simulink model "InverseKinematics_DirectionalController2018b"  (R2018b)
settings: Solver=VariableStepAuto  StartTime=0.0  StopTime=inf  RelTol=1e-3
undefined symbols (not defined in the file): f
libraries: instrumentlib x15, dspnetwork x6
(part 1 of 3)
settings Model: Creator=nisit  LastModifiedBy=Jskyl
settings DataIOCC: ReturnWorkspaceOutputs=on

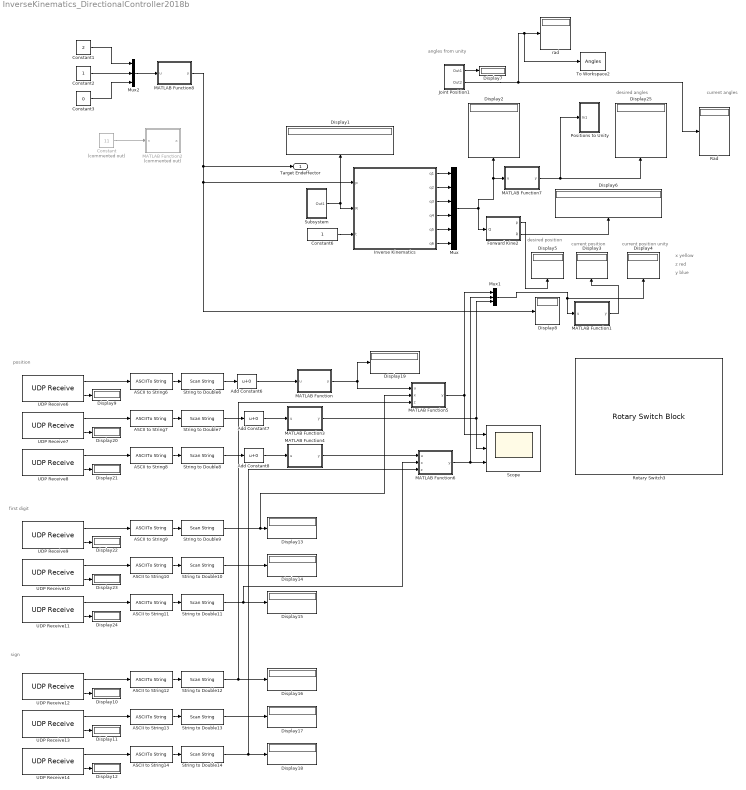
== system InverseKinematics_DirectionalController2018b ==
  note: angles from unity
  note: sign
  note: first digit
  note: position
  note: x yellow
  note: current position unity
  note: current position
  note: desired position
  note: current angles
  note: desired angles
  note: z red
  note: y blue
  ASCII to String{6..14} (9 alike) : ASCIIToString
  Add Constant6 : Bias
  Add Constant7 : Bias
  Add Constant8 : Bias
  Constant : Constant  Commented=on  Value=11
  Constant1 : Constant  Value=2
  Constant2 : Constant
  Constant3 : Constant  Value=0
  Constant6 : Constant
  Display{1..25} (25 alike) : Display
      Display10 settings: Format=bank
      Display11 settings: Format=bank
      Display12 settings: Format=bank
      Display20 settings: Format=bank
      Display21 settings: Format=bank
      Display22 settings: Format=bank
      Display23 settings: Format=bank
      Display24 settings: Format=bank
      Display9 settings: Format=bank
  Forward Kine2 : MATLAB Function  TreatAsAtomicUnit=on
  Inverse Kinematics : MATLAB Function  TreatAsAtomicUnit=on
  Joint Position1 : Subsystem
  MATLAB Function : MATLAB Function  TreatAsAtomicUnit=on
  MATLAB Function1 : MATLAB Function  TreatAsAtomicUnit=on
  MATLAB Function2 : MATLAB Function  Commented=on  TreatAsAtomicUnit=on
  MATLAB Function3 : MATLAB Function  TreatAsAtomicUnit=on
  MATLAB Function4 : MATLAB Function  TreatAsAtomicUnit=on
  MATLAB Function5 : MATLAB Function  TreatAsAtomicUnit=on
  MATLAB Function6 : MATLAB Function  TreatAsAtomicUnit=on
  MATLAB Function7 : MATLAB Function  TreatAsAtomicUnit=on
  MATLAB Function8 : MATLAB Function  TreatAsAtomicUnit=on
  Mux : Mux  Inputs=6
      settings: DisplayOption=signals
  Mux1 : Mux  Inputs=3
  Mux2 : Mux  Inputs=3
  Positions to Unity : Subsystem
  Rad : Display
  Rotary Switch3 : RotarySwitchBlock  WebBlockId=399
      settings: Values={{'Up', 'Down', 'In', 'out', 'Left', 'Right', 'Rest'}, [11 21 31 41 51 61 72]}
  Scope : Scope  NumInputPorts=3
  String to Double{6..14} (9 alike) : ScanString  Format="\"%lf\""
  Subsystem : Subsystem
  To Workspace2 : ToWorkspace  VariableName=Angles  SampleTime=-1
      settings: Save2DSignal=2-D array (concatenate along first dimension)
  UDP Receive10 : instrumentlib/UDP Receive  Host=localhost  Port=6200  LocalPort=6200  EnablePortSharing=off  GetLatestData=on  DataSize="[1  1]"  DataType=uint8  ASCIIFormatting=%f,  Terminator=LF  ByteOrder=BigEndian  EnableBlockingMode=off  Timeout=10  SampleTime=0.02  LocalAddress=127.0.0.1
  UDP Receive11 : instrumentlib/UDP Receive  Host=localhost  Port=6300  LocalPort=6300  EnablePortSharing=off  GetLatestData=on  DataSize="[1  1]"  DataType=uint8  ASCIIFormatting=%f,  Terminator=LF  ByteOrder=BigEndian  EnableBlockingMode=off  Timeout=10  SampleTime=0.02  LocalAddress=127.0.0.1
  UDP Receive12 : instrumentlib/UDP Receive  Host=localhost  Port=7100  LocalPort=7100  EnablePortSharing=off  GetLatestData=on  DataSize="[1  1]"  DataType=uint8  ASCIIFormatting=%f,  Terminator=LF  ByteOrder=BigEndian  EnableBlockingMode=off  Timeout=10  SampleTime=0.02  LocalAddress=127.0.0.1
  UDP Receive13 : instrumentlib/UDP Receive  Host=localhost  Port=7200  LocalPort=7200  EnablePortSharing=off  GetLatestData=on  DataSize="[1  1]"  DataType=uint8  ASCIIFormatting=%f,  Terminator=LF  ByteOrder=BigEndian  EnableBlockingMode=off  Timeout=10  SampleTime=0.02  LocalAddress=127.0.0.1
  UDP Receive14 : instrumentlib/UDP Receive  Host=localhost  Port=7300  LocalPort=7300  EnablePortSharing=off  GetLatestData=on  DataSize="[1  1]"  DataType=uint8  ASCIIFormatting=%f,  Terminator=LF  ByteOrder=BigEndian  EnableBlockingMode=off  Timeout=10  SampleTime=0.02  LocalAddress=127.0.0.1
  UDP Receive6 : instrumentlib/UDP Receive  Host=localhost  Port=5100  LocalPort=5100  EnablePortSharing=off  GetLatestData=on  DataSize="[1  7]"  DataType=uint8  ASCIIFormatting=%f,  Terminator=LF  ByteOrder=BigEndian  EnableBlockingMode=off  Timeout=10  SampleTime=0.02  LocalAddress=127.0.0.1
  UDP Receive7 : instrumentlib/UDP Receive  Host=localhost  Port=5200  LocalPort=5200  EnablePortSharing=off  GetLatestData=on  DataSize="[1  6]"  DataType=uint8  ASCIIFormatting=%f,  Terminator=LF  ByteOrder=BigEndian  EnableBlockingMode=off  Timeout=10  SampleTime=0.02  LocalAddress=127.0.0.1
  UDP Receive8 : instrumentlib/UDP Receive  Host=localhost  Port=5300  LocalPort=5300  EnablePortSharing=off  GetLatestData=on  DataSize="[1  7]"  DataType=uint8  ASCIIFormatting=%f,  Terminator=LF  ByteOrder=BigEndian  EnableBlockingMode=off  Timeout=10  SampleTime=0.02  LocalAddress=127.0.0.1
  UDP Receive9 : instrumentlib/UDP Receive  Host=localhost  Port=6100  LocalPort=6100  EnablePortSharing=off  GetLatestData=on  DataSize="[1  1]"  DataType=uint8  ASCIIFormatting=%f,  Terminator=LF  ByteOrder=BigEndian  EnableBlockingMode=off  Timeout=10  SampleTime=0.02  LocalAddress=127.0.0.1
  rad : Display
  Target Endeffector : Outport
  wires:
  Inverse Kinematics/1(q1) -> Mux/1
  Inverse Kinematics/2(q2) -> Mux/2
  Inverse Kinematics/3(q3) -> Mux/3
  Inverse Kinematics/4(q4) -> Mux/4
  Inverse Kinematics/5(q5) -> Mux/5
  Inverse Kinematics/6(q6) -> Mux/6
  Forward Kine2/1(p) -> Display5/1
  Forward Kine2/2(R) -> Display6/1
  Constant6/1 -> Inverse Kinematics/3(t)
  Mux/1 -> Display2/1, MATLAB Function7/1(u), Forward Kine2/1(Q)
  Joint Position1/2(Out2) -> To Workspace2/1, rad/1, Rad/1
  Joint Position1/1(Out1) -> Display7/1
  UDP Receive10/2 -> Display23/1
  MATLAB Function4/1(y) -> MATLAB Function6/1(u)
  String to Double12/1 -> Display16/1, MATLAB Function5/3(z)
  UDP Receive14/1 -> ASCII to String14/1
  String to Double11/1 -> MATLAB Function6/2(x), Display15/1
  UDP Receive9/2 -> Display22/1
  UDP Receive6/1 -> ASCII to String6/1
  UDP Receive12/2 -> Display10/1
  UDP Receive12/1 -> ASCII to String12/1
  ASCII to String12/1 -> String to Double12/1
  Add Constant6/1 -> MATLAB Function/1(u)
  ASCII to String8/1 -> String to Double8/1
  UDP Receive13/2 -> Display11/1
  ASCII to String14/1 -> String to Double14/1
  Add Constant7/1 -> MATLAB Function3/1(u)
  ASCII to String13/1 -> String to Double13/1
  MATLAB Function5/1(y) -> Scope/1, Mux1/1
  String to Double14/1 -> Display18/1, MATLAB Function6/3(z)
  UDP Receive14/2 -> Display12/1
  UDP Receive11/1 -> ASCII to String11/1
  String to Double10/1 -> Display14/1
  String to Double13/1 -> Display17/1
  ASCII to String7/1 -> String to Double7/1
  UDP Receive13/1 -> ASCII to String13/1
  UDP Receive10/1 -> ASCII to String10/1
  UDP Receive7/1 -> ASCII to String7/1
  UDP Receive8/2 -> Display21/1
  String to Double9/1 -> Display13/1, MATLAB Function5/2(x)
  ASCII to String9/1 -> String to Double9/1
  UDP Receive11/2 -> Display24/1
  MATLAB Function/1(y) -> Display19/1, MATLAB Function5/1(u)
  Add Constant8/1 -> MATLAB Function4/1(u)
  UDP Receive6/2 -> Display9/1
  MATLAB Function6/1(y) -> Scope/3, Mux1/2
  UDP Receive9/1 -> ASCII to String9/1
  UDP Receive8/1 -> ASCII to String8/1
  String to Double6/1 -> Add Constant6/1
  ASCII to String10/1 -> String to Double10/1
  UDP Receive7/2 -> Display20/1
  String to Double8/1 -> Add Constant8/1
  String to Double7/1 -> Add Constant7/1
  ASCII to String11/1 -> String to Double11/1
  ASCII to String6/1 -> String to Double6/1
  MATLAB Function3/1(y) -> Scope/2, Mux1/3
  Subsystem/1(Out1) -> Inverse Kinematics/2(R), Display1/1
  Mux1/1 -> MATLAB Function1/1(u), Display4/1
  MATLAB Function1/1(y) -> Display3/1
  MATLAB Function7/1(y) -> Positions to Unity/1(In1), Display25/1
  Constant1/1 -> Mux2/1
  Constant2/1 -> Mux2/2
  Constant3/1 -> Mux2/3
  Mux2/1 -> MATLAB Function8/1(u)
  MATLAB Function8/1(y) -> Inverse Kinematics/1(p), Display8/1, Target Endeffector/1
  Constant/1 -> MATLAB Function2/1(n)

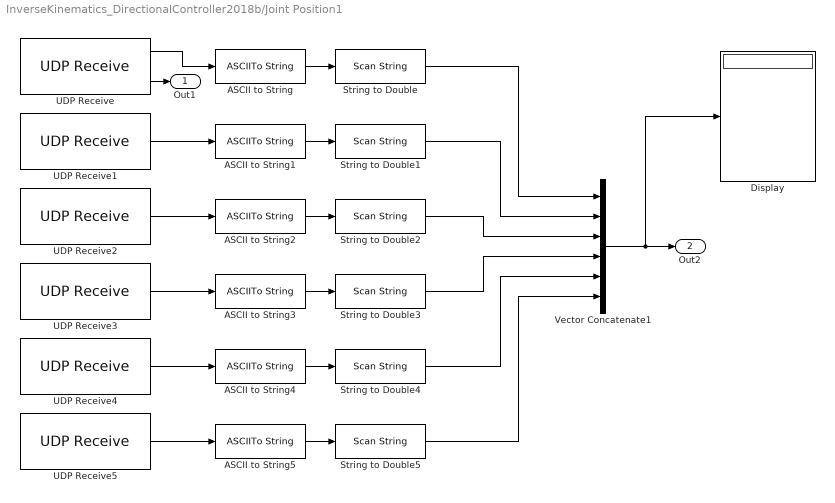
== system InverseKinematics_DirectionalController2018b/Joint Position1 ==
  ASCII to String{,1..5} (6 alike) : ASCIIToString
  Display : Display
  String to Double{,1..5} (6 alike) : ScanString  Format="\"%lf\""
  UDP Receive : instrumentlib/UDP Receive  Host=localhost  Port=2001  LocalPort=2001  EnablePortSharing=off  GetLatestData=off  DataSize="[5  1]"  DataType=uint8  ASCIIFormatting=%f,  Terminator=LF  ByteOrder=BigEndian  EnableBlockingMode=off  Timeout=10  SampleTime=0.01  LocalAddress=127.0.0.1
  UDP Receive1 : instrumentlib/UDP Receive  Host=localhost  Port=2002  LocalPort=2002  EnablePortSharing=off  GetLatestData=off  DataSize="[5  1]"  DataType=uint8  ASCIIFormatting=%f,  Terminator=LF  ByteOrder=BigEndian  EnableBlockingMode=on  Timeout=10  SampleTime=0.01  LocalAddress=127.0.0.1
  UDP Receive2 : instrumentlib/UDP Receive  Host=localhost  Port=2003  LocalPort=2003  EnablePortSharing=off  GetLatestData=off  DataSize="[5  1]"  DataType=uint8  ASCIIFormatting=%f,  Terminator=LF  ByteOrder=BigEndian  EnableBlockingMode=on  Timeout=10  SampleTime=0.01  LocalAddress=127.0.0.1
  UDP Receive3 : instrumentlib/UDP Receive  Host=localhost  Port=2004  LocalPort=2004  EnablePortSharing=off  GetLatestData=off  DataSize="[5  1]"  DataType=uint8  ASCIIFormatting=%f,  Terminator=LF  ByteOrder=BigEndian  EnableBlockingMode=on  Timeout=10  SampleTime=0.01  LocalAddress=127.0.0.1
  UDP Receive4 : instrumentlib/UDP Receive  Host=localhost  Port=2005  LocalPort=2005  EnablePortSharing=off  GetLatestData=off  DataSize="[5  1]"  DataType=uint8  ASCIIFormatting=%f,  Terminator=LF  ByteOrder=BigEndian  EnableBlockingMode=on  Timeout=10  SampleTime=0.01  LocalAddress=127.0.0.1
  UDP Receive5 : instrumentlib/UDP Receive  Host=localhost  Port=2006  LocalPort=2006  EnablePortSharing=off  GetLatestData=off  DataSize="[5  1]"  DataType=uint8  ASCIIFormatting=%f,  Terminator=LF  ByteOrder=BigEndian  EnableBlockingMode=on  Timeout=10  SampleTime=0.01  LocalAddress=127.0.0.1
  Vector Concatenate1 : Concatenate  NumInputs=6
  Out1 : Outport
  Out2 : Outport  Port=2
  wires:
  String to Double3/1 -> Vector Concatenate1/4
  String to Double4/1 -> Vector Concatenate1/5
  UDP Receive1/1 -> ASCII to String1/1
  String to Double1/1 -> Vector Concatenate1/2
  UDP Receive4/1 -> ASCII to String4/1
  UDP Receive3/1 -> ASCII to String3/1
  String to Double/1 -> Vector Concatenate1/1
  ASCII to String4/1 -> String to Double4/1
  String to Double2/1 -> Vector Concatenate1/3
  ASCII to String2/1 -> String to Double2/1
  ASCII to String3/1 -> String to Double3/1
  Vector Concatenate1/1 -> Display/1, Out2/1
  String to Double5/1 -> Vector Concatenate1/6
  ASCII to String1/1 -> String to Double1/1
  UDP Receive/1 -> ASCII to String/1
  UDP Receive5/1 -> ASCII to String5/1
  UDP Receive2/1 -> ASCII to String2/1
  ASCII to String5/1 -> String to Double5/1
  ASCII to String/1 -> String to Double/1
  UDP Receive/2 -> Out1/1

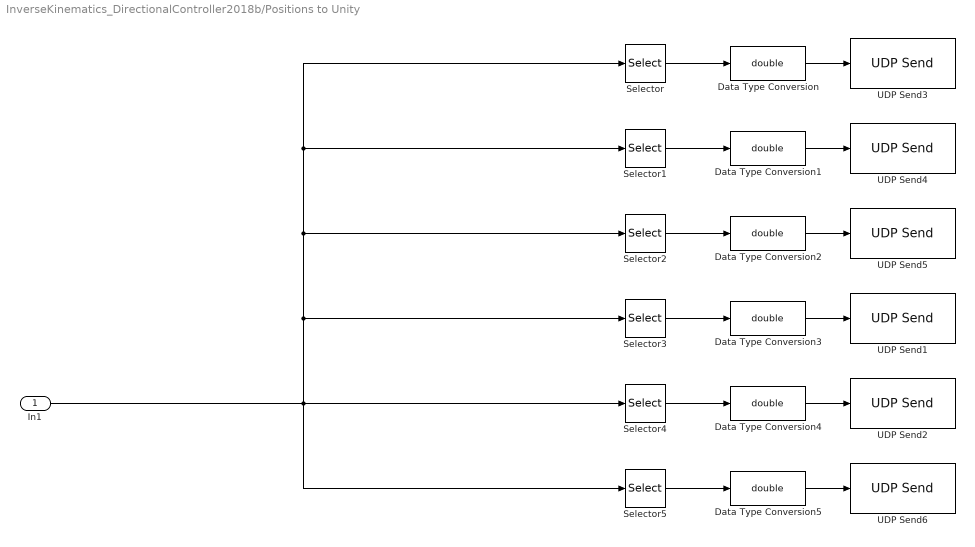
== system InverseKinematics_DirectionalController2018b/Positions to Unity ==
  In1 : Inport
  Data Type Conversion{,1..5} (6 alike) : DataTypeConversion  OutDataTypeStr=double  ConvertRealWorld=Stored Integer (SI)
  Selector : Selector  InputPortWidth=6  IndexOptions=Index vector (dialog)  Indices=[1]  OutputSizes=1
  Selector1 : Selector  InputPortWidth=6  IndexOptions=Index vector (dialog)  Indices=[2]  OutputSizes=1
  Selector2 : Selector  InputPortWidth=6  IndexOptions=Index vector (dialog)  Indices=[3]  OutputSizes=1
  Selector3 : Selector  InputPortWidth=6  IndexOptions=Index vector (dialog)  Indices=[4]  OutputSizes=1
  Selector4 : Selector  InputPortWidth=6  IndexOptions=Index vector (dialog)  Indices=[5]  OutputSizes=1
  Selector5 : Selector  InputPortWidth=6  IndexOptions=Index vector (dialog)  Indices=[6]  OutputSizes=1
  UDP Send1 : dspnetwork/UDP Send  remoteURL='127.0.0.1'  remotePort=3004  localURL='0.0.0.0'  localPortSource=Automatically determine  localPort=-1  sampletime=-1  blockPlatform=[]  separateLengthPort=0
  UDP Send2 : dspnetwork/UDP Send  remoteURL='127.0.0.1'  remotePort=3005  localURL='0.0.0.0'  localPortSource=Automatically determine  localPort=-1  sampletime=-1  blockPlatform=[]  separateLengthPort=0
  UDP Send3 : dspnetwork/UDP Send  remoteURL='127.0.0.1'  remotePort=3001  localURL='0.0.0.0'  localPortSource=Automatically determine  localPort=-1  sampletime=-1  blockPlatform=[]  separateLengthPort=0
  UDP Send4 : dspnetwork/UDP Send  remoteURL='127.0.0.1'  remotePort=3002  localURL='0.0.0.0'  localPortSource=Automatically determine  localPort=-1  sampletime=-1  blockPlatform=[]  separateLengthPort=0
  UDP Send5 : dspnetwork/UDP Send  remoteURL='127.0.0.1'  remotePort=3003  localURL='0.0.0.0'  localPortSource=Automatically determine  localPort=-1  sampletime=-1  blockPlatform=[]  separateLengthPort=0
  UDP Send6 : dspnetwork/UDP Send  remoteURL='127.0.0.1'  remotePort=3006  localURL='0.0.0.0'  localPortSource=Automatically determine  localPort=-1  sampletime=-1  blockPlatform=[]  separateLengthPort=0
  wires:
  Data Type Conversion2/1 -> UDP Send5/1
  Selector5/1 -> Data Type Conversion5/1
  In1/1 -> Selector/1, Selector1/1, Selector2/1, Selector3/1, Selector5/1, Selector4/1
  Selector2/1 -> Data Type Conversion2/1
  Data Type Conversion3/1 -> UDP Send1/1
  Data Type Conversion1/1 -> UDP Send4/1
  Data Type Conversion5/1 -> UDP Send6/1
  Selector1/1 -> Data Type Conversion1/1
  Selector4/1 -> Data Type Conversion4/1
  Selector3/1 -> Data Type Conversion3/1
  Data Type Conversion4/1 -> UDP Send2/1
  Selector/1 -> Data Type Conversion/1
  Data Type Conversion/1 -> UDP Send3/1

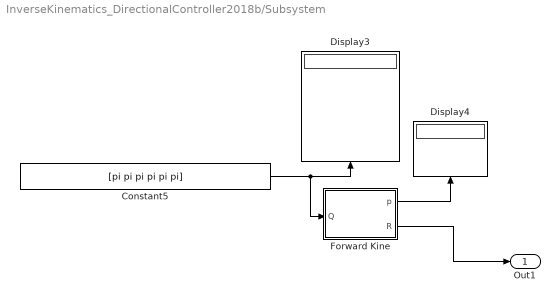
== system InverseKinematics_DirectionalController2018b/Subsystem ==
  Constant5 : Constant  Value=[pi pi pi pi pi pi]
  Display3 : Display
  Display4 : Display
  Forward Kine : MATLAB Function  TreatAsAtomicUnit=on
  Out1 : Outport
  wires:
  Constant5/1 -> Forward Kine/1(Q), Display3/1
  Forward Kine/1(p) -> Display4/1
  Forward Kine/2(R) -> Out1/1

== matlab function InverseKinematics_DirectionalController2018b/Forward Kine2 ==
  data: Q input; p output; R output
function [p,R] = fcn(Q)

%Inputs
Th_1=Q(1);
Th_2=Q(2);
Th_3=Q(3);
Th_4=Q(4);
Th_5=Q(5);
Th_6=Q(6);

% 
% Th_1=-1.6851;
% Th_2=-0.7011;
% Th_3=-3.3627;
% Th_4=0.3119;
% Th_5=1.7655;
% Th_6=-1.0709;

e2=0.0070;
D1=0.2755;
D2=0.2900;
D3=0.1233;
D4=0.0741;
D5=0.0741;
D6=0.1600;
aa=(30*pi)/180;
aa2=aa*2;
aa2d=rad2deg(aa2);
sa=sin(aa);
s2a=sin(2*aa);
d4b=D3+(sa/s2a)*D4;
d5b=(sa/s2a)*D4+(sa/s2a)*D5;
d6b=(sa/s2a)*D5 + D6;

%DH Table
a = [0;D2;0;0;0;0];
b = [D1;0;-e2;-d4b;-d5b; -d6b];
alpha = [90;180;90;aa2d;aa2d;180]*(pi/180);
%% Jaco Robot parameters based on the Forward Kinematic
% The following parameters are based on the paper Polynomial Inverse
% Kinematic Solution of the Jaco Robot. The below parameters can be
% % changed to meet the parameters of the Jaco Robot that we have at the lab.
% b__1 = 0.2755;  %Base to shoulder
% a__2 = 0.2900;  %Upper arm length (shoulder to elbow)
% b__3 = -0.0070; %Joint 3-4 lateral offset
% b__4 = -0.0741; %Distance from elbow to first sub-segment of the first wrist 
% %semgment
% b__5 = -0.0741; %Distance from end of the first sub-segment to of the first
% % wrist segment to end of the first sub-segment of the second wrist segment
% b__6 = -0.1600; % Distance from the end of the first sub-segment of the 
% % second wrist segment to the center of the hand.
% s__r4 = sind(55); %55 degrees is the angle of curvature first wrist segment
% s__r5 = sind(55); %55 degrees is the angle of curvature first wrist segment
% c__r4 = cosd(55); %55 degrees is the angle of curvature second wrist segment
% c__r5 = cosd(55); %55 degrees is the angle of curvature second wrist segment

%Function for Transformation Matrix 
A=@(theta,a,d,alpha) ([cos(theta),-sin(theta)*cos(alpha),sin(theta)*sin(alpha),a*cos(theta);sin(theta),cos(theta)*cos(alpha),-cos(theta)*sin(alpha),a*sin(theta);0,sin(alpha),cos(alpha),d;0,0,0,1]);

% Calculate the different A matrices and then calculate the DH matrix
A1 = A(Th_1,a(1),b(1),alpha(1));
A2 = A(Th_2,a(2),b(2),alpha(2));
A3 = A(Th_3,a(3),b(3),alpha(3));
A4 = A(Th_4,a(4),b(4),alpha(4));
A5 = A(Th_5,a(5),b(5),alpha(5));
A6 = A(Th_6,a(6),b(6),alpha(6));

%Transformation Matrix 
% T1=A1;
% T2=A1*A2;
% T3=A1*A2*A3;
% T4=A1*A2*A3*A4;
% T5=A1*A2*A3*A4*A5;
T6=A1*A2*A3*A4*A5*A6;

Ox = T6(1,4);
Oy = T6(2,4);
Oz = T6(3,4);
p=[Ox;Oy;Oz]

R=T6(1:3,1:3)

== matlab function InverseKinematics_DirectionalController2018b/Subsystem/Forward Kine ==
  data: Q input; p output; R output
function [p,R] = fcn(Q)

%Inputs
Th_1=Q(1);
Th_2=Q(2);
Th_3=Q(3);
Th_4=Q(4);
Th_5=Q(5);
Th_6=Q(6);

% 
% Th_1=-1.6851;
% Th_2=-0.7011;
% Th_3=-3.3627;
% Th_4=0.3119;
% Th_5=1.7655;
% Th_6=-1.0709;

e2=0.0070;
D1=0.2755;
D2=0.2900;
D3=0.1233;
D4=0.0741;
D5=0.0741;
D6=0.1600;
aa=(30*pi)/180;
aa2=aa*2;
aa2d=rad2deg(aa2);
sa=sin(aa);
s2a=sin(2*aa);
d4b=D3+(sa/s2a)*D4;
d5b=(sa/s2a)*D4+(sa/s2a)*D5;
d6b=(sa/s2a)*D5 + D6;

%DH Table
a = [0;D2;0;0;0;0];
b = [D1;0;-e2;-d4b;-d5b; -d6b];
alpha = [90;180;90;aa2d;aa2d;180]*(pi/180);
%% Jaco Robot parameters based on the Forward Kinematic
% The following parameters are based on the paper Polynomial Inverse
% Kinematic Solution of the Jaco Robot. The below parameters can be
% % changed to meet the parameters of the Jaco Robot that we have at the lab.
% b__1 = 0.2755;  %Base to shoulder
% a__2 = 0.2900;  %Upper arm length (shoulder to elbow)
% b__3 = -0.0070; %Joint 3-4 lateral offset
% b__4 = -0.0741; %Distance from elbow to first sub-segment of the first wrist 
% %semgment
% b__5 = -0.0741; %Distance from end of the first sub-segment to of the first
% % wrist segment to end of the first sub-segment of the second wrist segment
% b__6 = -0.1600; % Distance from the end of the first sub-segment of the 
% % second wrist segment to the center of the hand.
% s__r4 = sind(55); %55 degrees is the angle of curvature first wrist segment
% s__r5 = sind(55); %55 degrees is the angle of curvature first wrist segment
% c__r4 = cosd(55); %55 degrees is the angle of curvature second wrist segment
% c__r5 = cosd(55); %55 degrees is the angle of curvature second wrist segment

%Function for Transformation Matrix 
A=@(theta,a,d,alpha) ([cos(theta),-sin(theta)*cos(alpha),sin(theta)*sin(alpha),a*cos(theta);sin(theta),cos(theta)*cos(alpha),-cos(theta)*sin(alpha),a*sin(theta);0,sin(alpha),cos(alpha),d;0,0,0,1]);

% Calculate the different A matrices and then calculate the DH matrix
A1 = A(Th_1,a(1),b(1),alpha(1));
A2 = A(Th_2,a(2),b(2),alpha(2));
A3 = A(Th_3,a(3),b(3),alpha(3));
A4 = A(Th_4,a(4),b(4),alpha(4));
A5 = A(Th_5,a(5),b(5),alpha(5));
A6 = A(Th_6,a(6),b(6),alpha(6));

%Transformation Matrix 
% T1=A1;
% T2=A1*A2;
% T3=A1*A2*A3;
% T4=A1*A2*A3*A4;
% T5=A1*A2*A3*A4*A5;
T6=A1*A2*A3*A4*A5*A6;

Ox = T6(1,4);
Oy = T6(2,4);
Oz = T6(3,4);
p=[Ox;Oy;Oz]

R=T6(1:3,1:3)

== matlab function InverseKinematics_DirectionalController2018b/MATLAB Function2 ==
  data: n input; a output
function a = Pos(n)
% n = input('Enter a number: ');
  
switch n
  
    case 11
        a=[0.2,-0.1,-0.3]; % up
    case 21
        a=[-0.01,-0.1,-0.3]; % down
    case 31
        a=[0.2,0.27,-0.3]; % in
    case 41
        a=[0,0,0.1]; % out
    case 51
        a=[-0.2,0.1,-0.2]; % left
    case 61
        a=[0.2,-0.1,0.2]; % right
    case 71
        a=[0.2,-0.1,-0.3]; % rest
    otherwise
        a=[0.2,-0.1,-0.3]; % rest
end

% case 11
%         a=[0.15,-0.1,-0.3];
%     case 21
%         a=[0.10,-0.1,-0.3];
%     case 31
%         a=[0.2,-0.2,-0.3];
%     case 41
%         a=[0.2,0.1,-0.3];
%     case 51
%         a=[0.2,-0.1,-0.28];
%     case 61
%         a=[0.2,-0.1,-0.36];
%     case 71
%         a=[0.2,-0.1,-0.3];
%     otherwise
%         a=[0.2,-0.1,-0.3];

== matlab function InverseKinematics_DirectionalController2018b/MATLAB Function1 ==
  data: u input; y output
function y = fcn(u)

x = [u(1); -u(2); u(3)];
y = x/29;
%y = -t/29;
%y = z/29;

== matlab function InverseKinematics_DirectionalController2018b/MATLAB Function ==
  data: u input; y output
function y = fcn(u)

if u > 1
    c = sprintf('%f', u);
    y = str2double(c(2:6));
    %disp(y);
else
    y = u;
end

== matlab function InverseKinematics_DirectionalController2018b/MATLAB Function3 ==
  data: u input; y output
function y = fcn(u)

if u > 10
    c = sprintf('%f', u);
    y = str2double(c(2:6));
    disp(y);
else
    y = u;
end
